simulink model "JointFunctionalArch"  (R2024b)
settings: Solver=VariableStepAuto  StartTime=0.0  StopTime=10.0  RelTol=1e-3
settings Model: Creator=mfussi  LastModifiedBy=mfussi

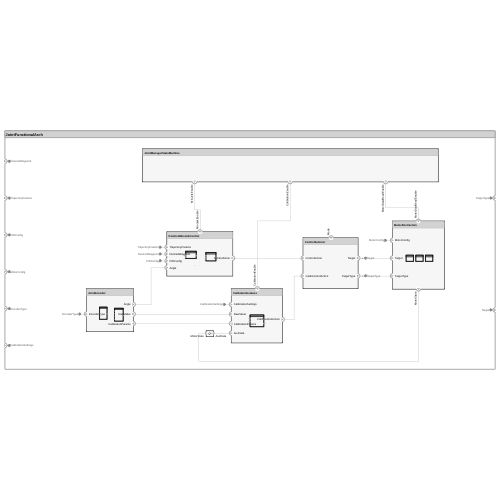
[thumbnail: Simulink's stored preview of the top-level diagram]
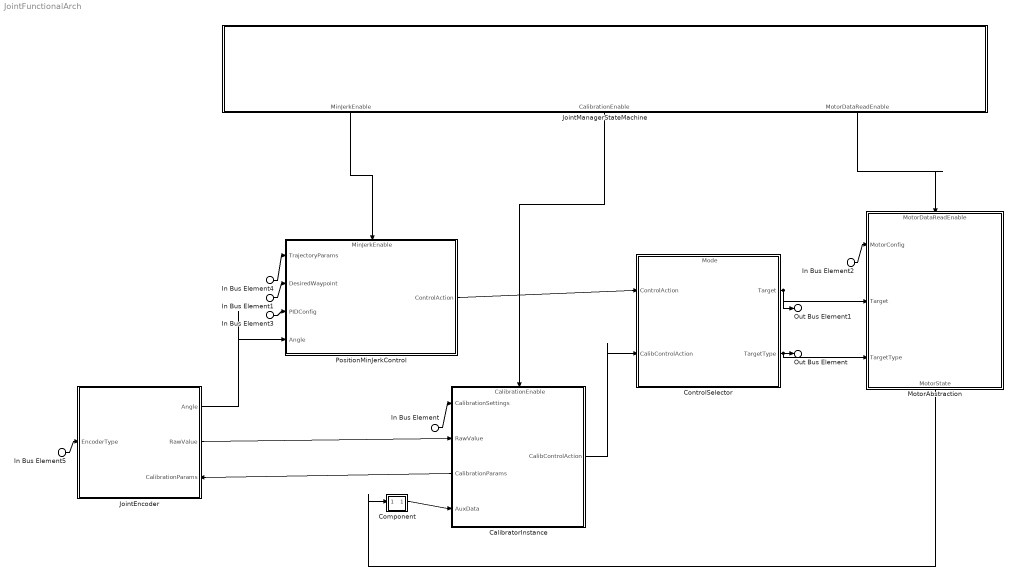
== system JointFunctionalArch ==
  In Bus Element1 : Inport  PortName=DesiredWaypoint
  In Bus Element4 : Inport  Port=2  PortName=TrajectoryParams
  In Bus Element3 : Inport  Port=3  PortName=PIDConfig
  In Bus Element2 : Inport  Port=4  PortName=MotorConfig
  In Bus Element5 : Inport  Port=5  PortName=EncoderType
  In Bus Element : Inport  Port=6  PortName=CalibrationSettings
  CalibratorInstance : Subsystem
      settings: PortSchema="{\"entries\":[{\"content\":{\"headerSize\":26,\"margin\":15,\"minimumSpacing\":25,\"sides\":[{\"content\":{\"connectorIds\":[\"In2\",\"In3\",\"Out1\",\"In4\"]},\"type\":\"ConnectorPlacement.EquallySpacedRectSide\",\"uuid\":\"01a9f67f-de41-4770-8c99-b8ecc5be53ce\"},{\"content\":{\"connectorIds\":[\"Out2\"],\"side\":\"RIGHT\"},\"type\":\"ConnectorPlacement.EquallySpacedRectSide\",\"uuid\":\"bf951eb2-be85-4331-ab1b-e1ec4c58de10\"},{\"content\":{\"connectorIds\":[\"In1\"],\"side\":\"TOP\"},\"type\":\"ConnectorPlacement.EquallySpacedRectSide\",\"uuid\":\"bda0090a-3dbc-4c35-be89-fb46a9401bc0\"},{\"content\":{\"side\":\"BOTTOM\"},\"type\":\"ConnectorPlacement.EquallySpacedRectSide\",\"uuid\":\"ec3dea10-cab4-440e-89eb-654eef2537c3\"}]},\"type\":\"ConnectorPlacement.EquallySpacedConnector\",\"uuid\":\"c83d3565-87fc-4d8e-ad9f-6c471e7c3840\"}],\"packageUris\":[\"http://schema.mathworks.com/mf0/Connector/R2020b\"],\"version\":\"1.0\"}"
  Component : Subsystem
      settings: PortSchema="{\"entries\":[{\"content\":{\"margin\":10,\"minimumSpacing\":15,\"sides\":[{\"content\":{\"connectorIds\":[\"In1\"]},\"type\":\"ConnectorPlacement.EquallySpacedRectSide\",\"uuid\":\"8e6109ac-b489-4864-8b2b-7ebf0beccfe4\"},{\"content\":{\"connectorIds\":[\"Out1\"],\"side\":\"RIGHT\"},\"type\":\"ConnectorPlacement.EquallySpacedRectSide\",\"uuid\":\"71828a7e-6b05-4f57-abc1-6f865453b9f6\"},{\"content\":{\"side\":\"TOP\"},\"type\":\"ConnectorPlacement.EquallySpacedRectSide\",\"uuid\":\"bfeeaaf9-6170-4b48-807f-b679c72692dc\"}]},\"type\":\"ConnectorPlacement.EquallySpacedConnector\",\"uuid\":\"352ed8e9-1880-4bea-97e7-a2aba6f573a0\"}],\"packageUris\":[\"http://schema.mathworks.com/mf0/Connector/R2020b\"],\"version\":\"1.0\"}"
  ControlSelector : Subsystem
      settings: PortSchema="{\"entries\":[{\"content\":{\"headerSize\":26,\"margin\":15,\"minimumSpacing\":25,\"sides\":[{\"content\":{\"connectorIds\":[\"In3\",\"In2\"]},\"type\":\"ConnectorPlacement.EquallySpacedRectSide\",\"uuid\":\"01a9f67f-de41-4770-8c99-b8ecc5be53ce\"},{\"content\":{\"connectorIds\":[\"Out1\",\"Out2\"],\"side\":\"RIGHT\"},\"type\":\"ConnectorPlacement.EquallySpacedRectSide\",\"uuid\":\"bf951eb2-be85-4331-ab1b-e1ec4c58de10\"},{\"content\":{\"connectorIds\":[\"In1\"],\"side\":\"TOP\"},\"type\":\"ConnectorPlacement.EquallySpacedRectSide\",\"uuid\":\"bda0090a-3dbc-4c35-be89-fb46a9401bc0\"}]},\"type\":\"ConnectorPlacement.EquallySpacedConnector\",\"uuid\":\"c83d3565-87fc-4d8e-ad9f-6c471e7c3840\"}],\"packageUris\":[\"http://schema.mathworks.com/mf0/Connector/R2020b\"],\"version\":\"1.0\"}"
  JointEncoder : Subsystem
      settings: PortSchema="{\"entries\":[{\"content\":{\"headerSize\":26,\"margin\":15,\"minimumSpacing\":25,\"sides\":[{\"content\":{\"connectorIds\":[\"In1\"]},\"type\":\"ConnectorPlacement.EquallySpacedRectSide\",\"uuid\":\"01a9f67f-de41-4770-8c99-b8ecc5be53ce\"},{\"content\":{\"connectorIds\":[\"Out2\",\"Out1\",\"In2\"],\"side\":\"RIGHT\"},\"type\":\"ConnectorPlacement.EquallySpacedRectSide\",\"uuid\":\"bf951eb2-be85-4331-ab1b-e1ec4c58de10\"},{\"content\":{\"side\":\"TOP\"},\"type\":\"ConnectorPlacement.EquallySpacedRectSide\",\"uuid\":\"bda0090a-3dbc-4c35-be89-fb46a9401bc0\"},{\"content\":{\"side\":\"BOTTOM\"},\"type\":\"ConnectorPlacement.EquallySpacedRectSide\",\"uuid\":\"08402c68-e81a-4e51-a9bb-186315986595\"}]},\"type\":\"ConnectorPlacement.EquallySpacedConnector\",\"uuid\":\"c83d3565-87fc-4d8e-ad9f-6c471e7c3840\"}],\"packageUris\":[\"http://schema.mathworks.com/mf0/Connector/R2020b\"],\"version\":\"1.0\"}"
  JointManagerStateMachine : Subsystem
      settings: PortSchema="{\"entries\":[{\"content\":{\"headerSize\":26,\"margin\":15,\"minimumSpacing\":25,\"sides\":[{\"content\":{},\"type\":\"ConnectorPlacement.EquallySpacedRectSide\",\"uuid\":\"8e6109ac-b489-4864-8b2b-7ebf0beccfe4\"},{\"content\":{\"side\":\"RIGHT\"},\"type\":\"ConnectorPlacement.EquallySpacedRectSide\",\"uuid\":\"71828a7e-6b05-4f57-abc1-6f865453b9f6\"},{\"content\":{\"side\":\"TOP\"},\"type\":\"ConnectorPlacement.EquallySpacedRectSide\",\"uuid\":\"bfeeaaf9-6170-4b48-807f-b679c72692dc\"},{\"content\":{\"connectorIds\":[\"Out1\",\"Out2\",\"Out3\"],\"side\":\"BOTTOM\"},\"type\":\"ConnectorPlacement.EquallySpacedRectSide\",\"uuid\":\"8d96d7f2-73a1-4d5a-99fb-90680abef3dc\"}]},\"type\":\"ConnectorPlacement.EquallySpacedConnector\",\"uuid\":\"352ed8e9-1880-4bea-97e7-a2aba6f573a0\"}],\"packageUris\":[\"http://schema.mathworks.com/mf0/Connector/R2020b\"],\"version\":\"1.0\"}"
  MotorAbstraction : Subsystem
      settings: PortSchema="{\"entries\":[{\"content\":{\"headerSize\":26,\"margin\":15,\"minimumSpacing\":25,\"sides\":[{\"content\":{\"connectorIds\":[\"In2\",\"In3\",\"In4\"]},\"type\":\"ConnectorPlacement.EquallySpacedRectSide\",\"uuid\":\"01a9f67f-de41-4770-8c99-b8ecc5be53ce\"},{\"content\":{\"side\":\"RIGHT\"},\"type\":\"ConnectorPlacement.EquallySpacedRectSide\",\"uuid\":\"bf951eb2-be85-4331-ab1b-e1ec4c58de10\"},{\"content\":{\"connectorIds\":[\"In1\"],\"side\":\"TOP\"},\"type\":\"ConnectorPlacement.EquallySpacedRectSide\",\"uuid\":\"bda0090a-3dbc-4c35-be89-fb46a9401bc0\"},{\"content\":{\"connectorIds\":[\"Out1\"],\"side\":\"BOTTOM\"},\"type\":\"ConnectorPlacement.EquallySpacedRectSide\",\"uuid\":\"213d38af-1bfb-4ede-ab92-b167cd142b13\"}]},\"type\":\"ConnectorPlacement.EquallySpacedConnector\",\"uuid\":\"c83d3565-87fc-4d8e-ad9f-6c471e7c3840\"}],\"packageUris\":[\"http://schema.mathworks.com/mf0/Connector/R2020b\"],\"version\":\"1.0\"}"
  PositionMinJerkControl : Subsystem
      settings: PortSchema="{\"entries\":[{\"content\":{\"headerSize\":26,\"margin\":15,\"minimumSpacing\":25,\"sides\":[{\"content\":{\"connectorIds\":[\"In2\",\"In3\",\"In4\",\"In5\"]},\"type\":\"ConnectorPlacement.EquallySpacedRectSide\",\"uuid\":\"a6b52f4d-c0be-425e-a602-92486203cf1a\"},{\"content\":{\"connectorIds\":[\"Out1\"],\"side\":\"RIGHT\"},\"type\":\"ConnectorPlacement.EquallySpacedRectSide\",\"uuid\":\"97de3152-cc67-4140-b6b8-81845a876737\"},{\"content\":{\"connectorIds\":[\"In1\"],\"side\":\"TOP\"},\"type\":\"ConnectorPlacement.EquallySpacedRectSide\",\"uuid\":\"ebc405a6-c557-4a2e-ab17-42ca9b397efe\"}]},\"type\":\"ConnectorPlacement.EquallySpacedConnector\",\"uuid\":\"3652fe7f-5812-4192-9520-9c06c6702b26\"}],\"packageUris\":[\"http://schema.mathworks.com/mf0/Connector/R2020b\"],\"version\":\"1.0\"}"
  Out Bus Element : Outport  PortName=TargetType
  Out Bus Element1 : Outport  Port=2  PortName=Target
  wires:
  CalibratorInstance/2(CalibControlAction) -> ControlSelector/2(CalibControlAction)
  JointEncoder/1(RawValue) -> CalibratorInstance/3(RawValue)
  CalibratorInstance/1(CalibrationParams) -> JointEncoder/2(CalibrationParams)
  ControlSelector/2(TargetType) -> Out Bus Element/1, MotorAbstraction/4(TargetType)
  In Bus Element/1 -> CalibratorInstance/2(CalibrationSettings)
  In Bus Element2/1 -> MotorAbstraction/2(MotorConfig)
  ControlSelector/1(Target) -> Out Bus Element1/1, MotorAbstraction/3(Target)
  Component/1(AuxData) -> CalibratorInstance/4(AuxData)
  MotorAbstraction/1(MotorState) -> Component/1(MotorState)
  In Bus Element5/1 -> JointEncoder/1(EncoderType)
  In Bus Element4/1 -> PositionMinJerkControl/2(TrajectoryParams)
  In Bus Element1/1 -> PositionMinJerkControl/3(DesiredWaypoint)
  In Bus Element3/1 -> PositionMinJerkControl/4(PIDConfig)
  JointEncoder/2(Angle) -> PositionMinJerkControl/5(Angle)
  PositionMinJerkControl/1(ControlAction) -> ControlSelector/3(ControlAction)
  JointManagerStateMachine/1(MinJerkEnable) -> PositionMinJerkControl/1(MinJerkEnable)
  JointManagerStateMachine/3(MotorDataReadEnable) -> MotorAbstraction/1(MotorDataReadEnable)
  JointManagerStateMachine/2(CalibrationEnable) -> CalibratorInstance/1(CalibrationEnable)

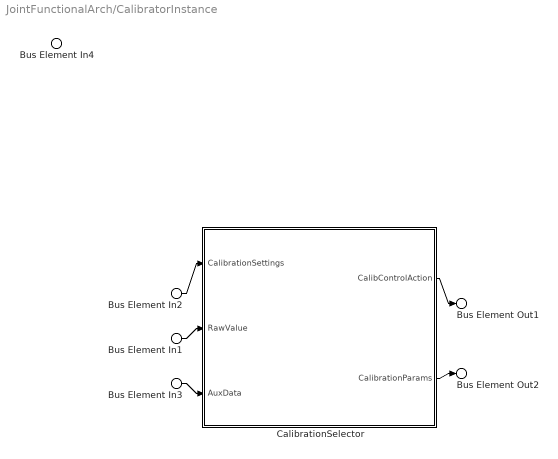
== system JointFunctionalArch/CalibratorInstance ==
  Bus Element In4 : Inport  PortName=CalibrationEnable
  Bus Element In2 : Inport  Port=2  PortName=CalibrationSettings
  Bus Element In1 : Inport  Port=3  PortName=RawValue
  Bus Element In3 : Inport  Port=4  PortName=AuxData
  CalibrationSelector : Subsystem
      settings: PortSchema="{\"entries\":[{\"content\":{\"headerSize\":26,\"margin\":15,\"minimumSpacing\":25,\"sides\":[{\"content\":{\"connectorIds\":[\"In2\",\"In3\",\"In1\"]},\"type\":\"ConnectorPlacement.EquallySpacedRectSide\",\"uuid\":\"8e6109ac-b489-4864-8b2b-7ebf0beccfe4\"},{\"content\":{\"connectorIds\":[\"Out1\",\"Out2\"],\"side\":\"RIGHT\"},\"type\":\"ConnectorPlacement.EquallySpacedRectSide\",\"uuid\":\"71828a7e-6b05-4f57-abc1-6f865453b9f6\"},{\"content\":{\"side\":\"TOP\"},\"type\":\"ConnectorPlacement.EquallySpacedRectSide\",\"uuid\":\"bfeeaaf9-6170-4b48-807f-b679c72692dc\"},{\"content\":{\"side\":\"BOTTOM\"},\"type\":\"ConnectorPlacement.EquallySpacedRectSide\",\"uuid\":\"25c92704-7839-4043-9d29-39ffe7db8a81\"}]},\"type\":\"ConnectorPlacement.EquallySpacedConnector\",\"uuid\":\"352ed8e9-1880-4bea-97e7-a2aba6f573a0\"}],\"packageUris\":[\"http://schema.mathworks.com/mf0/Connector/R2020b\"],\"version\":\"1.0\"}"
  Bus Element Out2 : Outport  PortName=CalibrationParams
  Bus Element Out1 : Outport  Port=2  PortName=CalibControlAction
  wires:
  Bus Element In2/1 -> CalibrationSelector/2(CalibrationSettings)
  CalibrationSelector/2(CalibrationParams) -> Bus Element Out2/1
  Bus Element In1/1 -> CalibrationSelector/3(RawValue)
  Bus Element In3/1 -> CalibrationSelector/1(AuxData)
  CalibrationSelector/1(CalibControlAction) -> Bus Element Out1/1

== system JointFunctionalArch/Component ==
  In Bus Element : Inport  PortName=MotorState
  Out Bus Element : Outport  PortName=AuxData
  wires:
  In Bus Element/1 -> Out Bus Element/1

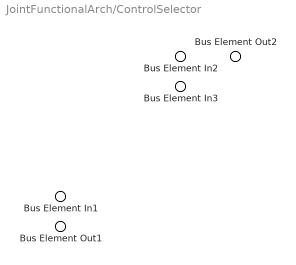
== system JointFunctionalArch/ControlSelector ==
  Bus Element In3 : Inport  PortName=Mode
  Bus Element In2 : Inport  Port=2  PortName=CalibControlAction
  Bus Element In1 : Inport  Port=3  PortName=ControlAction
  Bus Element Out2 : Outport  PortName=Target
  Bus Element Out1 : Outport  Port=2  PortName=TargetType

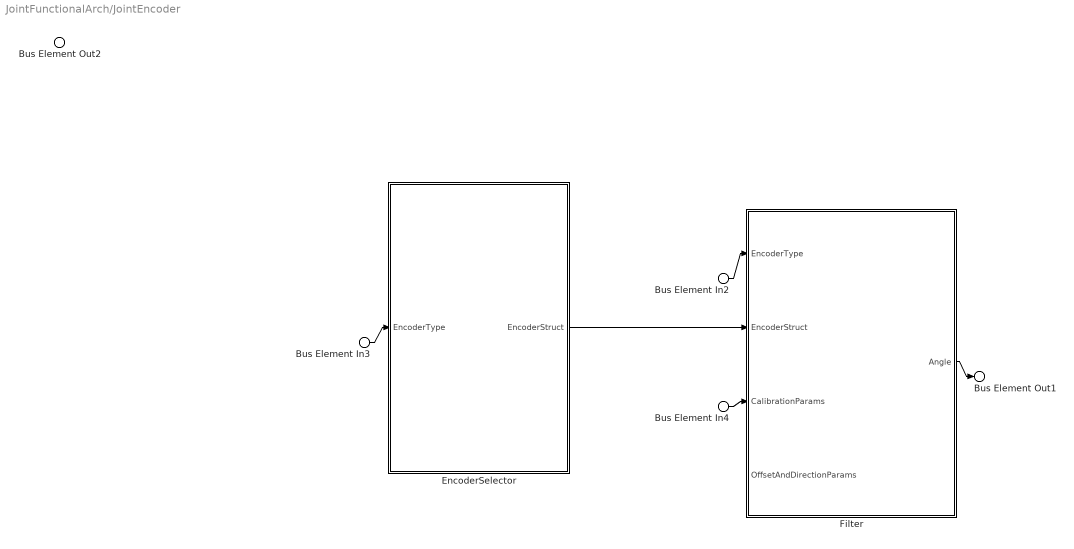
== system JointFunctionalArch/JointEncoder ==
  Bus Element In2 : Inport  PortName=EncoderType
  Bus Element In3 : Inport  PortName=EncoderType
  Bus Element In4 : Inport  Port=2  PortName=CalibrationParams
  EncoderSelector : Subsystem
      settings: PortSchema="{\"entries\":[{\"content\":{\"headerSize\":26,\"margin\":15,\"minimumSpacing\":25,\"sides\":[{\"content\":{\"connectorIds\":[\"In1\"]},\"type\":\"ConnectorPlacement.EquallySpacedRectSide\",\"uuid\":\"8f52fc44-033b-42c5-ba74-e10c3c4c9620\"},{\"content\":{\"connectorIds\":[\"Out1\"],\"side\":\"RIGHT\"},\"type\":\"ConnectorPlacement.EquallySpacedRectSide\",\"uuid\":\"3378411c-333a-4ac7-97cd-fc73e032020d\"},{\"content\":{\"side\":\"TOP\"},\"type\":\"ConnectorPlacement.EquallySpacedRectSide\",\"uuid\":\"71f34e7e-b8af-4493-b4da-76896ccc3fbc\"}]},\"type\":\"ConnectorPlacement.EquallySpacedConnector\",\"uuid\":\"3896a3b2-2849-4eb4-a68e-00b6690583b8\"}],\"packageUris\":[\"http://schema.mathworks.com/mf0/Connector/R2020b\"],\"version\":\"1.0\"}"
  Filter : Subsystem
      settings: PortSchema="{\"entries\":[{\"content\":{\"headerSize\":26,\"margin\":15,\"minimumSpacing\":25,\"sides\":[{\"content\":{\"connectorIds\":[\"In3\",\"In2\",\"In4\",\"In1\"]},\"type\":\"ConnectorPlacement.EquallySpacedRectSide\",\"uuid\":\"8e6109ac-b489-4864-8b2b-7ebf0beccfe4\"},{\"content\":{\"connectorIds\":[\"Out1\"],\"side\":\"RIGHT\"},\"type\":\"ConnectorPlacement.EquallySpacedRectSide\",\"uuid\":\"71828a7e-6b05-4f57-abc1-6f865453b9f6\"},{\"content\":{\"side\":\"TOP\"},\"type\":\"ConnectorPlacement.EquallySpacedRectSide\",\"uuid\":\"bfeeaaf9-6170-4b48-807f-b679c72692dc\"},{\"content\":{\"side\":\"BOTTOM\"},\"type\":\"ConnectorPlacement.EquallySpacedRectSide\",\"uuid\":\"712cf681-e2bb-4a2f-a437-e98f589a9711\"}]},\"type\":\"ConnectorPlacement.EquallySpacedConnector\",\"uuid\":\"352ed8e9-1880-4bea-97e7-a2aba6f573a0\"}],\"packageUris\":[\"http://schema.mathworks.com/mf0/Connector/R2020b\"],\"version\":\"1.0\"}"
  Bus Element Out2 : Outport  PortName=RawValue
  Bus Element Out1 : Outport  Port=2  PortName=Angle
  wires:
  Filter/1(Angle) -> Bus Element Out1/1
  Bus Element In2/1 -> Filter/3(EncoderType)
  Bus Element In3/1 -> EncoderSelector/1(EncoderType)
  EncoderSelector/1(EncoderStruct) -> Filter/2(EncoderStruct)
  Bus Element In4/1 -> Filter/4(CalibrationParams)

== system JointFunctionalArch/JointManagerStateMachine ==
  Bus Element Out1 : Outport  PortName=MinJerkEnable
  Bus Element Out3 : Outport  Port=2  PortName=CalibrationEnable
  Bus Element Out2 : Outport  Port=3  PortName=MotorDataReadEnable

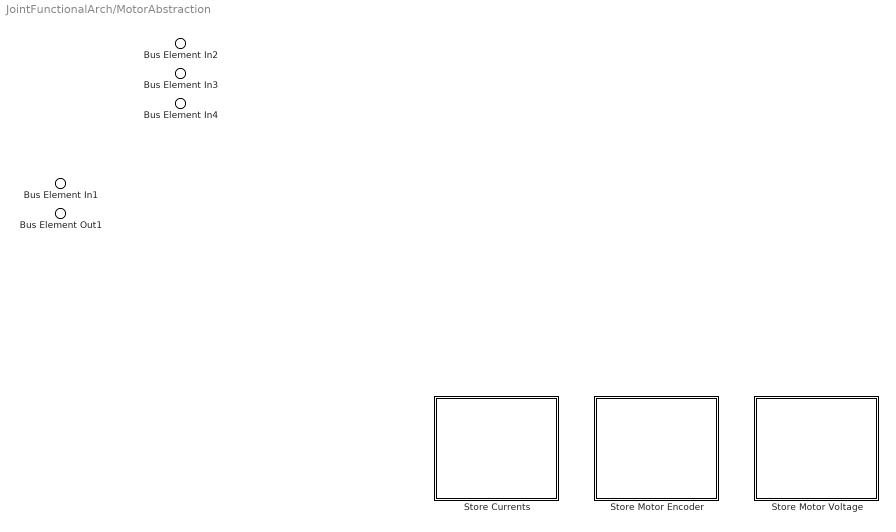
== system JointFunctionalArch/MotorAbstraction ==
  Bus Element In4 : Inport  PortName=MotorDataReadEnable
  Bus Element In2 : Inport  Port=2  PortName=MotorConfig
  Bus Element In3 : Inport  Port=3  PortName=Target
  Bus Element In1 : Inport  Port=4  PortName=TargetType
  Store Currents : Subsystem
      settings: PortSchema="{\"entries\":[{\"content\":{\"headerSize\":26,\"margin\":15,\"minimumSpacing\":25,\"sides\":[{\"content\":{},\"type\":\"ConnectorPlacement.EquallySpacedRectSide\",\"uuid\":\"8e6109ac-b489-4864-8b2b-7ebf0beccfe4\"},{\"content\":{\"side\":\"RIGHT\"},\"type\":\"ConnectorPlacement.EquallySpacedRectSide\",\"uuid\":\"71828a7e-6b05-4f57-abc1-6f865453b9f6\"},{\"content\":{\"side\":\"TOP\"},\"type\":\"ConnectorPlacement.EquallySpacedRectSide\",\"uuid\":\"bfeeaaf9-6170-4b48-807f-b679c72692dc\"}]},\"type\":\"ConnectorPlacement.EquallySpacedConnector\",\"uuid\":\"352ed8e9-1880-4bea-97e7-a2aba6f573a0\"}],\"packageUris\":[\"http://schema.mathworks.com/mf0/Connector/R2020b\"],\"version\":\"1.0\"}"
  Store Motor Encoder : Subsystem
      settings: PortSchema="{\"entries\":[{\"content\":{\"headerSize\":26,\"margin\":15,\"minimumSpacing\":25,\"sides\":[{\"content\":{},\"type\":\"ConnectorPlacement.EquallySpacedRectSide\",\"uuid\":\"8e6109ac-b489-4864-8b2b-7ebf0beccfe4\"},{\"content\":{\"side\":\"RIGHT\"},\"type\":\"ConnectorPlacement.EquallySpacedRectSide\",\"uuid\":\"71828a7e-6b05-4f57-abc1-6f865453b9f6\"},{\"content\":{\"side\":\"TOP\"},\"type\":\"ConnectorPlacement.EquallySpacedRectSide\",\"uuid\":\"bfeeaaf9-6170-4b48-807f-b679c72692dc\"}]},\"type\":\"ConnectorPlacement.EquallySpacedConnector\",\"uuid\":\"352ed8e9-1880-4bea-97e7-a2aba6f573a0\"}],\"packageUris\":[\"http://schema.mathworks.com/mf0/Connector/R2020b\"],\"version\":\"1.0\"}"
  Store Motor Voltage : Subsystem
      settings: PortSchema="{\"entries\":[{\"content\":{\"headerSize\":26,\"margin\":15,\"minimumSpacing\":25,\"sides\":[{\"content\":{},\"type\":\"ConnectorPlacement.EquallySpacedRectSide\",\"uuid\":\"8e6109ac-b489-4864-8b2b-7ebf0beccfe4\"},{\"content\":{\"side\":\"RIGHT\"},\"type\":\"ConnectorPlacement.EquallySpacedRectSide\",\"uuid\":\"71828a7e-6b05-4f57-abc1-6f865453b9f6\"},{\"content\":{\"side\":\"TOP\"},\"type\":\"ConnectorPlacement.EquallySpacedRectSide\",\"uuid\":\"bfeeaaf9-6170-4b48-807f-b679c72692dc\"}]},\"type\":\"ConnectorPlacement.EquallySpacedConnector\",\"uuid\":\"352ed8e9-1880-4bea-97e7-a2aba6f573a0\"}],\"packageUris\":[\"http://schema.mathworks.com/mf0/Connector/R2020b\"],\"version\":\"1.0\"}"
  Bus Element Out1 : Outport  PortName=MotorState

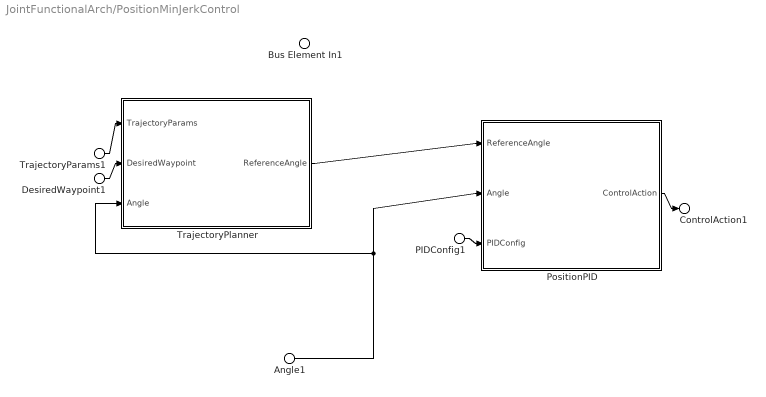
== system JointFunctionalArch/PositionMinJerkControl ==
  Bus Element In1 : Inport  PortName=MinJerkEnable
  TrajectoryParams1 : Inport  Port=2  PortName=TrajectoryParams
  DesiredWaypoint1 : Inport  Port=3  PortName=DesiredWaypoint
  PIDConfig1 : Inport  Port=4  PortName=PIDConfig
  Angle1 : Inport  Port=5  PortName=Angle
  PositionPID : Subsystem
      settings: PortSchema="{\"entries\":[{\"content\":{\"headerSize\":26,\"margin\":15,\"minimumSpacing\":25,\"sides\":[{\"content\":{\"connectorIds\":[\"In1\",\"In2\",\"In3\"]},\"type\":\"ConnectorPlacement.EquallySpacedRectSide\",\"uuid\":\"01a9f67f-de41-4770-8c99-b8ecc5be53ce\"},{\"content\":{\"connectorIds\":[\"Out1\"],\"side\":\"RIGHT\"},\"type\":\"ConnectorPlacement.EquallySpacedRectSide\",\"uuid\":\"bf951eb2-be85-4331-ab1b-e1ec4c58de10\"},{\"content\":{\"side\":\"TOP\"},\"type\":\"ConnectorPlacement.EquallySpacedRectSide\",\"uuid\":\"bda0090a-3dbc-4c35-be89-fb46a9401bc0\"},{\"content\":{\"side\":\"BOTTOM\"},\"type\":\"ConnectorPlacement.EquallySpacedRectSide\",\"uuid\":\"a00fa0d9-dee8-49f3-9b32-dc66d4ded2f3\"}]},\"type\":\"ConnectorPlacement.EquallySpacedConnector\",\"uuid\":\"c83d3565-87fc-4d8e-ad9f-6c471e7c3840\"}],\"packageUris\":[\"http://schema.mathworks.com/mf0/Connector/R2020b\"],\"version\":\"1.0\"}"
  TrajectoryPlanner : Subsystem
      settings: PortSchema="{\"entries\":[{\"content\":{\"headerSize\":26,\"margin\":15,\"minimumSpacing\":25,\"sides\":[{\"content\":{\"connectorIds\":[\"In1\",\"In2\",\"In3\"]},\"type\":\"ConnectorPlacement.EquallySpacedRectSide\",\"uuid\":\"01a9f67f-de41-4770-8c99-b8ecc5be53ce\"},{\"content\":{\"connectorIds\":[\"Out1\"],\"side\":\"RIGHT\"},\"type\":\"ConnectorPlacement.EquallySpacedRectSide\",\"uuid\":\"bf951eb2-be85-4331-ab1b-e1ec4c58de10\"},{\"content\":{\"side\":\"TOP\"},\"type\":\"ConnectorPlacement.EquallySpacedRectSide\",\"uuid\":\"bda0090a-3dbc-4c35-be89-fb46a9401bc0\"},{\"content\":{\"side\":\"BOTTOM\"},\"type\":\"ConnectorPlacement.EquallySpacedRectSide\",\"uuid\":\"b81b6dc1-9499-4eb9-b7d6-7b63466e4081\"}]},\"type\":\"ConnectorPlacement.EquallySpacedConnector\",\"uuid\":\"c83d3565-87fc-4d8e-ad9f-6c471e7c3840\"}],\"packageUris\":[\"http://schema.mathworks.com/mf0/Connector/R2020b\"],\"version\":\"1.0\"}"
  ControlAction1 : Outport  PortName=ControlAction
  wires:
  PIDConfig1/1 -> PositionPID/3(PIDConfig)
  TrajectoryParams1/1 -> TrajectoryPlanner/1(TrajectoryParams)
  TrajectoryPlanner/1(ReferenceAngle) -> PositionPID/1(ReferenceAngle)
  PositionPID/1(ControlAction) -> ControlAction1/1
  Angle1/1 -> TrajectoryPlanner/3(Angle), PositionPID/2(Angle)
  DesiredWaypoint1/1 -> TrajectoryPlanner/2(DesiredWaypoint)

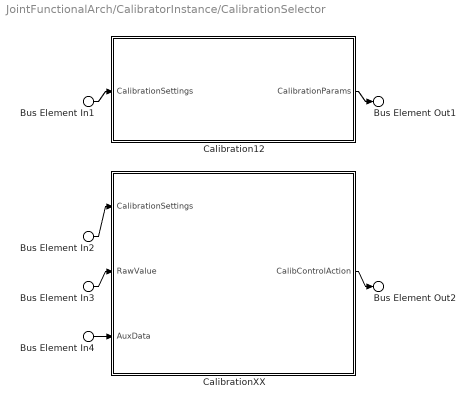
== system JointFunctionalArch/CalibratorInstance/CalibrationSelector ==
  Bus Element In4 : Inport  PortName=AuxData
  Bus Element In1 : Inport  Port=2  PortName=CalibrationSettings
  Bus Element In2 : Inport  Port=2  PortName=CalibrationSettings
  Bus Element In3 : Inport  Port=3  PortName=RawValue
  Calibration12 : Subsystem
      settings: PortSchema="{\"entries\":[{\"content\":{\"headerSize\":26,\"margin\":15,\"minimumSpacing\":25,\"sides\":[{\"content\":{\"connectorIds\":[\"In1\"]},\"type\":\"ConnectorPlacement.EquallySpacedRectSide\",\"uuid\":\"8e6109ac-b489-4864-8b2b-7ebf0beccfe4\"},{\"content\":{\"connectorIds\":[\"Out1\"],\"side\":\"RIGHT\"},\"type\":\"ConnectorPlacement.EquallySpacedRectSide\",\"uuid\":\"71828a7e-6b05-4f57-abc1-6f865453b9f6\"},{\"content\":{\"side\":\"TOP\"},\"type\":\"ConnectorPlacement.EquallySpacedRectSide\",\"uuid\":\"bfeeaaf9-6170-4b48-807f-b679c72692dc\"}]},\"type\":\"ConnectorPlacement.EquallySpacedConnector\",\"uuid\":\"352ed8e9-1880-4bea-97e7-a2aba6f573a0\"}],\"packageUris\":[\"http://schema.mathworks.com/mf0/Connector/R2020b\"],\"version\":\"1.0\"}"
  CalibrationXX : Subsystem
      settings: PortSchema="{\"entries\":[{\"content\":{\"headerSize\":26,\"margin\":15,\"minimumSpacing\":25,\"sides\":[{\"content\":{\"connectorIds\":[\"In1\",\"In2\",\"In3\"]},\"type\":\"ConnectorPlacement.EquallySpacedRectSide\",\"uuid\":\"8e6109ac-b489-4864-8b2b-7ebf0beccfe4\"},{\"content\":{\"connectorIds\":[\"Out1\"],\"side\":\"RIGHT\"},\"type\":\"ConnectorPlacement.EquallySpacedRectSide\",\"uuid\":\"71828a7e-6b05-4f57-abc1-6f865453b9f6\"},{\"content\":{\"side\":\"TOP\"},\"type\":\"ConnectorPlacement.EquallySpacedRectSide\",\"uuid\":\"bfeeaaf9-6170-4b48-807f-b679c72692dc\"},{\"content\":{\"side\":\"BOTTOM\"},\"type\":\"ConnectorPlacement.EquallySpacedRectSide\",\"uuid\":\"376d2493-7fe7-4dcb-93f0-7b1cd430ade4\"}]},\"type\":\"ConnectorPlacement.EquallySpacedConnector\",\"uuid\":\"352ed8e9-1880-4bea-97e7-a2aba6f573a0\"}],\"packageUris\":[\"http://schema.mathworks.com/mf0/Connector/R2020b\"],\"version\":\"1.0\"}"
  Bus Element Out2 : Outport  PortName=CalibControlAction
  Bus Element Out1 : Outport  Port=2  PortName=CalibrationParams
  wires:
  Bus Element In1/1 -> Calibration12/1(CalibrationSettings)
  Calibration12/1(CalibrationParams) -> Bus Element Out1/1
  Bus Element In2/1 -> CalibrationXX/1(CalibrationSettings)
  Bus Element In3/1 -> CalibrationXX/2(RawValue)
  Bus Element In4/1 -> CalibrationXX/3(AuxData)
  CalibrationXX/1(CalibControlAction) -> Bus Element Out2/1

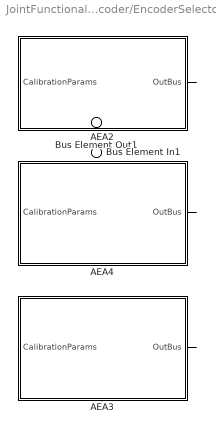
== system JointFunctionalArch/JointEncoder/EncoderSelector ==
  Bus Element In1 : Inport  PortName=EncoderType
  AEA2 : Subsystem
      settings: PortSchema="{\"entries\":[{\"content\":{\"headerSize\":26,\"margin\":15,\"minimumSpacing\":25,\"sides\":[{\"content\":{\"connectorIds\":[\"In1\"]},\"type\":\"ConnectorPlacement.EquallySpacedRectSide\",\"uuid\":\"8e6109ac-b489-4864-8b2b-7ebf0beccfe4\"},{\"content\":{\"connectorIds\":[\"Out1\"],\"side\":\"RIGHT\"},\"type\":\"ConnectorPlacement.EquallySpacedRectSide\",\"uuid\":\"71828a7e-6b05-4f57-abc1-6f865453b9f6\"},{\"content\":{\"side\":\"TOP\"},\"type\":\"ConnectorPlacement.EquallySpacedRectSide\",\"uuid\":\"bfeeaaf9-6170-4b48-807f-b679c72692dc\"}]},\"type\":\"ConnectorPlacement.EquallySpacedConnector\",\"uuid\":\"352ed8e9-1880-4bea-97e7-a2aba6f573a0\"}],\"packageUris\":[\"http://schema.mathworks.com/mf0/Connector/R2020b\"],\"version\":\"1.0\"}"
  AEA3 : Subsystem
      settings: PortSchema="{\"entries\":[{\"content\":{\"headerSize\":26,\"margin\":15,\"minimumSpacing\":25,\"sides\":[{\"content\":{\"connectorIds\":[\"In1\"]},\"type\":\"ConnectorPlacement.EquallySpacedRectSide\",\"uuid\":\"8e6109ac-b489-4864-8b2b-7ebf0beccfe4\"},{\"content\":{\"connectorIds\":[\"Out1\"],\"side\":\"RIGHT\"},\"type\":\"ConnectorPlacement.EquallySpacedRectSide\",\"uuid\":\"71828a7e-6b05-4f57-abc1-6f865453b9f6\"},{\"content\":{\"side\":\"TOP\"},\"type\":\"ConnectorPlacement.EquallySpacedRectSide\",\"uuid\":\"bfeeaaf9-6170-4b48-807f-b679c72692dc\"},{\"content\":{\"side\":\"BOTTOM\"},\"type\":\"ConnectorPlacement.EquallySpacedRectSide\",\"uuid\":\"a15bd14f-14b1-4784-ba04-128ef95cb1ea\"}]},\"type\":\"ConnectorPlacement.EquallySpacedConnector\",\"uuid\":\"352ed8e9-1880-4bea-97e7-a2aba6f573a0\"}],\"packageUris\":[\"http://schema.mathworks.com/mf0/Connector/R2020b\"],\"version\":\"1.0\"}"
  AEA4 : Subsystem
      settings: PortSchema="{\"entries\":[{\"content\":{\"headerSize\":26,\"margin\":15,\"minimumSpacing\":25,\"sides\":[{\"content\":{\"connectorIds\":[\"In1\"]},\"type\":\"ConnectorPlacement.EquallySpacedRectSide\",\"uuid\":\"8e6109ac-b489-4864-8b2b-7ebf0beccfe4\"},{\"content\":{\"connectorIds\":[\"Out1\"],\"side\":\"RIGHT\"},\"type\":\"ConnectorPlacement.EquallySpacedRectSide\",\"uuid\":\"71828a7e-6b05-4f57-abc1-6f865453b9f6\"},{\"content\":{\"side\":\"TOP\"},\"type\":\"ConnectorPlacement.EquallySpacedRectSide\",\"uuid\":\"bfeeaaf9-6170-4b48-807f-b679c72692dc\"},{\"content\":{\"side\":\"BOTTOM\"},\"type\":\"ConnectorPlacement.EquallySpacedRectSide\",\"uuid\":\"a15bd14f-14b1-4784-ba04-128ef95cb1ea\"}]},\"type\":\"ConnectorPlacement.EquallySpacedConnector\",\"uuid\":\"352ed8e9-1880-4bea-97e7-a2aba6f573a0\"}],\"packageUris\":[\"http://schema.mathworks.com/mf0/Connector/R2020b\"],\"version\":\"1.0\"}"
  Bus Element Out1 : Outport  PortName=EncoderStruct
  wires:
  AEA3/1(OutBus) -> ?
  AEA2/1(OutBus) -> ?
  AEA4/1(OutBus) -> ?

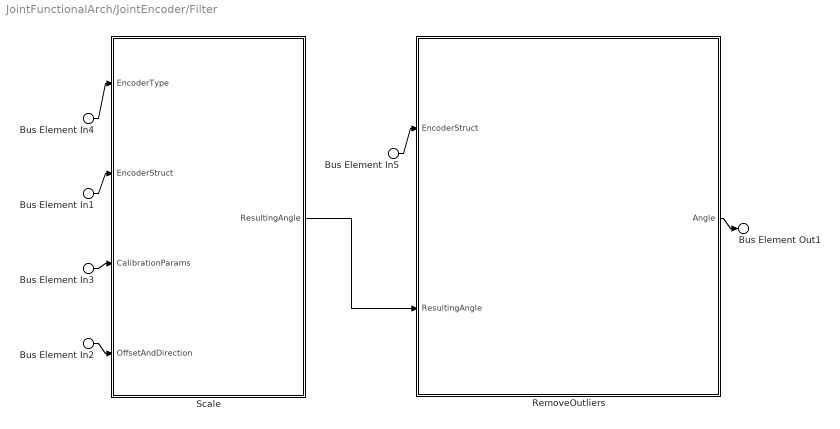
== system JointFunctionalArch/JointEncoder/Filter ==
  Bus Element In2 : Inport  PortName=OffsetAndDirectionParams
  Bus Element In1 : Inport  Port=2  PortName=EncoderStruct
  Bus Element In5 : Inport  Port=2  PortName=EncoderStruct
  Bus Element In4 : Inport  Port=3  PortName=EncoderType
  Bus Element In3 : Inport  Port=4  PortName=CalibrationParams
  RemoveOutliers : Subsystem
      settings: PortSchema="{\"entries\":[{\"content\":{\"headerSize\":26,\"margin\":15,\"minimumSpacing\":25,\"sides\":[{\"content\":{\"connectorIds\":[\"In1\",\"In2\"]},\"type\":\"ConnectorPlacement.EquallySpacedRectSide\",\"uuid\":\"8e6109ac-b489-4864-8b2b-7ebf0beccfe4\"},{\"content\":{\"connectorIds\":[\"Out1\"],\"side\":\"RIGHT\"},\"type\":\"ConnectorPlacement.EquallySpacedRectSide\",\"uuid\":\"71828a7e-6b05-4f57-abc1-6f865453b9f6\"},{\"content\":{\"side\":\"TOP\"},\"type\":\"ConnectorPlacement.EquallySpacedRectSide\",\"uuid\":\"bfeeaaf9-6170-4b48-807f-b679c72692dc\"}]},\"type\":\"ConnectorPlacement.EquallySpacedConnector\",\"uuid\":\"352ed8e9-1880-4bea-97e7-a2aba6f573a0\"}],\"packageUris\":[\"http://schema.mathworks.com/mf0/Connector/R2020b\"],\"version\":\"1.0\"}"
  Scale : Subsystem
      settings: PortSchema="{\"entries\":[{\"content\":{\"headerSize\":26,\"margin\":15,\"minimumSpacing\":25,\"sides\":[{\"content\":{\"connectorIds\":[\"In1\",\"In2\",\"In3\",\"In4\"]},\"type\":\"ConnectorPlacement.EquallySpacedRectSide\",\"uuid\":\"8e6109ac-b489-4864-8b2b-7ebf0beccfe4\"},{\"content\":{\"connectorIds\":[\"Out1\"],\"side\":\"RIGHT\"},\"type\":\"ConnectorPlacement.EquallySpacedRectSide\",\"uuid\":\"71828a7e-6b05-4f57-abc1-6f865453b9f6\"},{\"content\":{\"side\":\"TOP\"},\"type\":\"ConnectorPlacement.EquallySpacedRectSide\",\"uuid\":\"bfeeaaf9-6170-4b48-807f-b679c72692dc\"}]},\"type\":\"ConnectorPlacement.EquallySpacedConnector\",\"uuid\":\"352ed8e9-1880-4bea-97e7-a2aba6f573a0\"}],\"packageUris\":[\"http://schema.mathworks.com/mf0/Connector/R2020b\"],\"version\":\"1.0\"}"
  Bus Element Out1 : Outport  PortName=Angle
  wires:
  Bus Element In4/1 -> Scale/1(EncoderType)
  Bus Element In3/1 -> Scale/3(CalibrationParams)
  Bus Element In2/1 -> Scale/4(OffsetAndDirection)
  RemoveOutliers/1(Angle) -> Bus Element Out1/1
  Bus Element In1/1 -> Scale/2(EncoderStruct)
  Bus Element In5/1 -> RemoveOutliers/1(EncoderStruct)
  Scale/1(ResultingAngle) -> RemoveOutliers/2(ResultingAngle)

== system JointFunctionalArch/MotorAbstraction/Store Currents ==

== system JointFunctionalArch/MotorAbstraction/Store Motor Encoder ==

== system JointFunctionalArch/MotorAbstraction/Store Motor Voltage ==

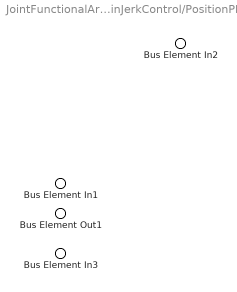
== system JointFunctionalArch/PositionMinJerkControl/PositionPID ==
  Bus Element In2 : Inport  PortName=ReferenceAngle
  Bus Element In1 : Inport  Port=2  PortName=Angle
  Bus Element In3 : Inport  Port=3  PortName=PIDConfig
  Bus Element Out1 : Outport  PortName=ControlAction

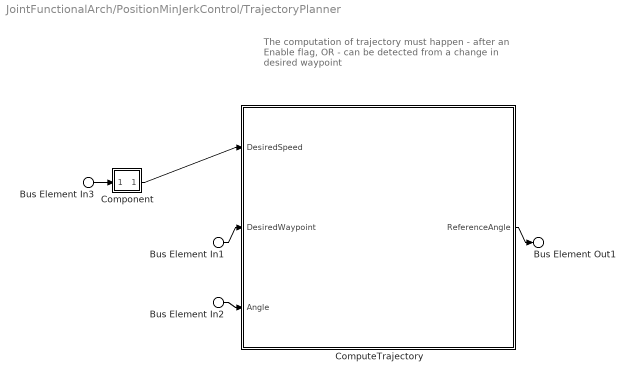
== system JointFunctionalArch/PositionMinJerkControl/TrajectoryPlanner ==
  note: The computation of trajectory must happen
      | - after an Enable flag, OR
      | - can be detected from a change in desired waypoint
  Bus Element In3 : Inport  PortName=TrajectoryParams
  Bus Element In1 : Inport  Port=2  PortName=DesiredWaypoint
  Bus Element In2 : Inport  Port=3  PortName=Angle
  Component : Subsystem
      settings: PortSchema="{\"entries\":[{\"content\":{\"margin\":10,\"minimumSpacing\":15,\"sides\":[{\"content\":{\"connectorIds\":[\"In1\"]},\"type\":\"ConnectorPlacement.EquallySpacedRectSide\",\"uuid\":\"8e6109ac-b489-4864-8b2b-7ebf0beccfe4\"},{\"content\":{\"connectorIds\":[\"Out1\"],\"side\":\"RIGHT\"},\"type\":\"ConnectorPlacement.EquallySpacedRectSide\",\"uuid\":\"71828a7e-6b05-4f57-abc1-6f865453b9f6\"},{\"content\":{\"side\":\"TOP\"},\"type\":\"ConnectorPlacement.EquallySpacedRectSide\",\"uuid\":\"bfeeaaf9-6170-4b48-807f-b679c72692dc\"}]},\"type\":\"ConnectorPlacement.EquallySpacedConnector\",\"uuid\":\"352ed8e9-1880-4bea-97e7-a2aba6f573a0\"}],\"packageUris\":[\"http://schema.mathworks.com/mf0/Connector/R2020b\"],\"version\":\"1.0\"}"
  ComputeTrajectory : Subsystem
      settings: PortSchema="{\"entries\":[{\"content\":{\"headerSize\":26,\"margin\":15,\"minimumSpacing\":25,\"sides\":[{\"content\":{\"connectorIds\":[\"In1\",\"In2\",\"In3\"]},\"type\":\"ConnectorPlacement.EquallySpacedRectSide\",\"uuid\":\"8e6109ac-b489-4864-8b2b-7ebf0beccfe4\"},{\"content\":{\"connectorIds\":[\"Out1\"],\"side\":\"RIGHT\"},\"type\":\"ConnectorPlacement.EquallySpacedRectSide\",\"uuid\":\"71828a7e-6b05-4f57-abc1-6f865453b9f6\"},{\"content\":{\"side\":\"TOP\"},\"type\":\"ConnectorPlacement.EquallySpacedRectSide\",\"uuid\":\"bfeeaaf9-6170-4b48-807f-b679c72692dc\"}]},\"type\":\"ConnectorPlacement.EquallySpacedConnector\",\"uuid\":\"352ed8e9-1880-4bea-97e7-a2aba6f573a0\"}],\"packageUris\":[\"http://schema.mathworks.com/mf0/Connector/R2020b\"],\"version\":\"1.0\"}"
  Bus Element Out1 : Outport  PortName=ReferenceAngle
  wires:
  Component/1(DesiredSpeed) -> ComputeTrajectory/1(DesiredSpeed)
  Bus Element In3/1 -> Component/1(TrajectoryParams)
  Bus Element In1/1 -> ComputeTrajectory/2(DesiredWaypoint)
  Bus Element In2/1 -> ComputeTrajectory/3(Angle)
  ComputeTrajectory/1(ReferenceAngle) -> Bus Element Out1/1

== system JointFunctionalArch/CalibratorInstance/CalibrationSelector/Calibration12 ==
  Bus Element In1 : Inport  PortName=CalibrationSettings
  Bus Element Out1 : Outport  PortName=CalibrationParams

== system JointFunctionalArch/CalibratorInstance/CalibrationSelector/CalibrationXX ==
  Bus Element In1 : Inport  PortName=CalibrationSettings
  Bus Element In2 : Inport  Port=2  PortName=RawValue
  Bus Element In3 : Inport  Port=3  PortName=AuxData
  Bus Element Out1 : Outport  PortName=CalibControlAction

== system JointFunctionalArch/JointEncoder/EncoderSelector/AEA2 ==
  Bus Element In1 : Inport  PortName=CalibrationParams
  Bus Element Out1 : Outport  PortName=OutBus

== system JointFunctionalArch/JointEncoder/EncoderSelector/AEA3 ==
  Bus Element In1 : Inport  PortName=CalibrationParams
  Bus Element Out1 : Outport  PortName=OutBus

== system JointFunctionalArch/JointEncoder/EncoderSelector/AEA4 ==
  Bus Element In1 : Inport  PortName=CalibrationParams
  Bus Element Out1 : Outport  PortName=OutBus

== system JointFunctionalArch/JointEncoder/Filter/RemoveOutliers ==
  Bus Element In1 : Inport  PortName=EncoderStruct
  Bus Element In2 : Inport  Port=2  PortName=ResultingAngle
  Bus Element Out1 : Outport  PortName=Angle

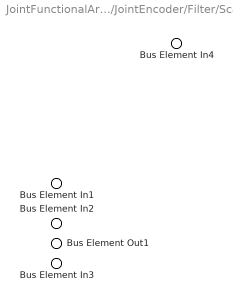
== system JointFunctionalArch/JointEncoder/Filter/Scale ==
  Bus Element In1 : Inport  PortName=EncoderType
  Bus Element In4 : Inport  Port=2  PortName=EncoderStruct
  Bus Element In2 : Inport  Port=3  PortName=CalibrationParams
  Bus Element In3 : Inport  Port=4  PortName=OffsetAndDirection
  Bus Element Out1 : Outport  PortName=ResultingAngle

== system JointFunctionalArch/PositionMinJerkControl/TrajectoryPlanner/Component ==
  In Bus Element : Inport  PortName=TrajectoryParams
  Out Bus Element : Outport  PortName=DesiredSpeed
  wires:
  In Bus Element/1 -> Out Bus Element/1

== system JointFunctionalArch/PositionMinJerkControl/TrajectoryPlanner/ComputeTrajectory ==
  Bus Element In1 : Inport  PortName=DesiredSpeed
  Bus Element In2 : Inport  Port=2  PortName=DesiredWaypoint
  Bus Element In3 : Inport  Port=3  PortName=Angle
  Bus Element Out1 : Outport  PortName=ReferenceAngle
